simulink model "P2"  (R2020a)
settings: Solver=VariableStepAuto  StartTime=0.0  StopTime=2000  RelTol=1e-3
undefined symbols (not defined in the file): Qin_1, Qin_2
libraries: cstblocks x2
settings Model: Creator=beto1  LastModifiedBy=beto1

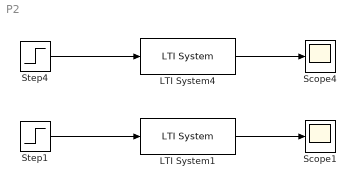
== system P2 ==
  LTI System1 : cstblocks/LTI System  sys=H2  IC=[]
  LTI System4 : cstblocks/LTI System  sys=H1  IC=[]
  Scope1 : Scope
  Scope4 : Scope
  Step1 : Step  Time=0  After=Qin_2  SampleTime=0
  Step4 : Step  Time=0  After=Qin_1  SampleTime=0
  wires:
  Step4/1 -> LTI System4/1
  LTI System4/1 -> Scope4/1
  Step1/1 -> LTI System1/1
  LTI System1/1 -> Scope1/1
